simulink library "mympclib"  (R2020a)
settings: Solver=VariableStepAuto  StartTime=0.0  StopTime=10.0  RelTol=1e-3
undefined symbols (not defined in the file): params, sysm, Ts
(part 2 of 2)

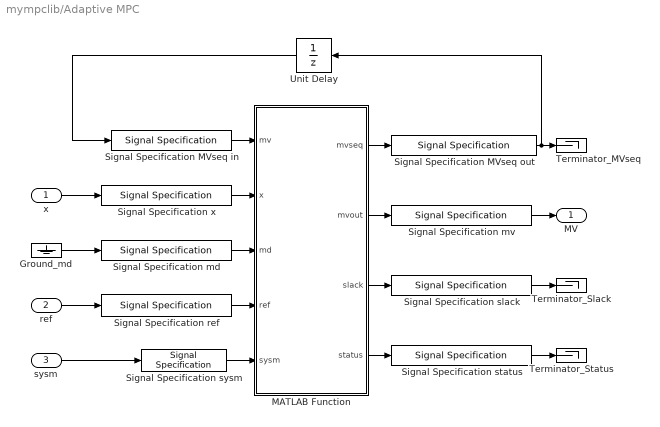
== system mympclib/Adaptive MPC ==
  x : Inport
  ref : Inport  Port=2
  sysm : Inport  Port=3
  Ground_md : Ground
  MATLAB Function : MATLAB Function  TreatAsAtomicUnit=on  SystemSampleTime=Ts
  Signal Specification MVseq in : SignalSpecification  OutDataTypeStr=double  Dimensions=index2  SampleTime=Ts
  Signal Specification MVseq out : SignalSpecification  OutDataTypeStr=double  Dimensions=index2  SampleTime=Ts
  Signal Specification md : SignalSpecification  OutDataTypeStr=double  Dimensions=numDist  SampleTime=Ts
  Signal Specification mv : SignalSpecification  OutDataTypeStr=double  Dimensions=numMV  SampleTime=Ts
  Signal Specification ref : SignalSpecification  OutDataTypeStr=double  Dimensions=numRef  SampleTime=Ts
  Signal Specification slack : SignalSpecification  OutDataTypeStr=double  Dimensions=1  SampleTime=Ts
  Signal Specification status : SignalSpecification  OutDataTypeStr=boolean  Dimensions=1  SampleTime=Ts
  Signal Specification sysm : SignalSpecification  SampleTime=Ts
  Signal Specification x : SignalSpecification  OutDataTypeStr=double  Dimensions=numState  SampleTime=Ts
  Terminator_MVseq : Terminator
  Terminator_Slack : Terminator
  Terminator_Status : Terminator
  Unit Delay : UnitDelay  InitialCondition=kron(ones(params.ControlHorizon,1) , params.initialconditionMV)  SampleTime=-1  HasFrameUpgradeWarning=on
  MV : Outport
  wires:
  MATLAB Function/3(slack) -> Signal Specification slack/1
  MATLAB Function/4(status) -> Signal Specification status/1
  x/1 -> Signal Specification x/1
  ref/1 -> Signal Specification ref/1
  Signal Specification x/1 -> MATLAB Function/2(x)
  Signal Specification md/1 -> MATLAB Function/3(md)
  Signal Specification ref/1 -> MATLAB Function/4(ref)
  sysm/1 -> Signal Specification sysm/1
  MATLAB Function/2(mvout) -> Signal Specification mv/1
  Signal Specification sysm/1 -> MATLAB Function/5(sysm)
  MATLAB Function/1(mvseq) -> Signal Specification MVseq out/1
  Unit Delay/1 -> Signal Specification MVseq in/1
  Signal Specification mv/1 -> MV/1
  Signal Specification MVseq in/1 -> MATLAB Function/1(mv)
  Signal Specification MVseq out/1 -> Unit Delay/1, Terminator_MVseq/1
  Signal Specification slack/1 -> Terminator_Slack/1
  Signal Specification status/1 -> Terminator_Status/1
  Ground_md/1 -> Signal Specification md/1

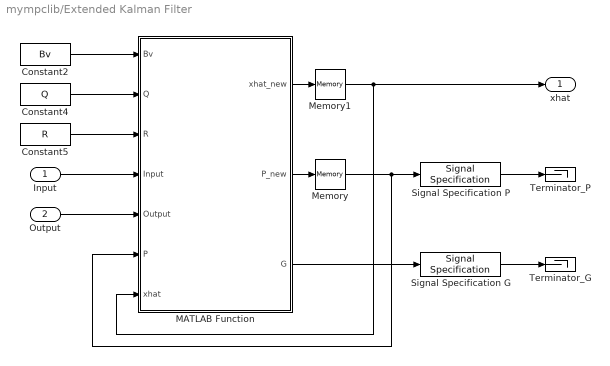
== system mympclib/Extended Kalman Filter ==
  Input : Inport
  Output : Inport  Port=2
  Constant2 : Constant  Value=Bv
  Constant4 : Constant  Value=Q
  Constant5 : Constant  Value=R
  MATLAB Function : MATLAB Function  TreatAsAtomicUnit=on  SystemSampleTime=Ts
  Memory : Memory  InitialCondition=P0  InheritSampleTime=on  LinearizeMemory=on  LinearizeAsDelay=on
  Memory1 : Memory  InitialCondition=xhat0  InheritSampleTime=on  LinearizeMemory=on  LinearizeAsDelay=on
  Signal Specification G : SignalSpecification  SampleTime=Ts
  Signal Specification P : SignalSpecification  SampleTime=Ts
  Terminator_G : Terminator
  Terminator_P : Terminator
  xhat : Outport
  wires:
  Constant2/1 -> MATLAB Function/1(Bv)
  MATLAB Function/3(G) -> Signal Specification G/1
  Constant5/1 -> MATLAB Function/3(R)
  Memory1/1 -> xhat/1, MATLAB Function/7(xhat)
  MATLAB Function/2(P_new) -> Memory/1
  MATLAB Function/1(xhat_new) -> Memory1/1
  Input/1 -> MATLAB Function/4(Input)
  Output/1 -> MATLAB Function/5(Output)
  Constant4/1 -> MATLAB Function/2(Q)
  Memory/1 -> Signal Specification P/1, MATLAB Function/6(P)
  Signal Specification P/1 -> Terminator_P/1
  Signal Specification G/1 -> Terminator_G/1

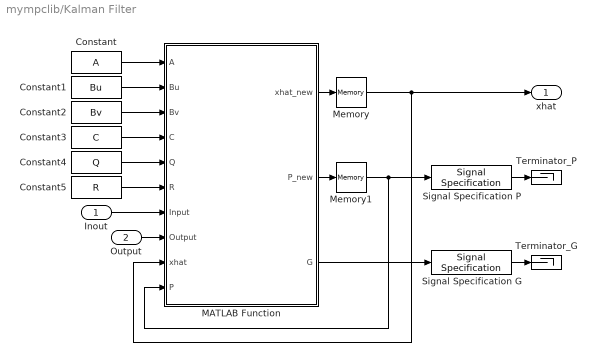
== system mympclib/Kalman Filter ==
  Inout : Inport
  Output : Inport  Port=2
  Constant : Constant  Value=A
  Constant1 : Constant  Value=Bu
  Constant2 : Constant  Value=Bv
  Constant3 : Constant  Value=C
  Constant4 : Constant  Value=Q
  Constant5 : Constant  Value=R
  MATLAB Function : MATLAB Function  TreatAsAtomicUnit=on  SystemSampleTime=Ts
  Memory : Memory  InitialCondition=xhat0  InheritSampleTime=on  LinearizeMemory=on  LinearizeAsDelay=on
  Memory1 : Memory  InitialCondition=P0  InheritSampleTime=on  LinearizeMemory=on  LinearizeAsDelay=on
  Signal Specification G : SignalSpecification  SampleTime=Ts
  Signal Specification P : SignalSpecification  SampleTime=Ts
  Terminator_G : Terminator
  Terminator_P : Terminator
  xhat : Outport
  wires:
  MATLAB Function/3(G) -> Signal Specification G/1
  Constant1/1 -> MATLAB Function/2(Bu)
  MATLAB Function/2(P_new) -> Memory1/1
  MATLAB Function/1(xhat_new) -> Memory/1
  Constant5/1 -> MATLAB Function/6(R)
  Inout/1 -> MATLAB Function/7(Input)
  Constant2/1 -> MATLAB Function/3(Bv)
  Constant3/1 -> MATLAB Function/4(C)
  Constant/1 -> MATLAB Function/1(A)
  Output/1 -> MATLAB Function/8(Output)
  Constant4/1 -> MATLAB Function/5(Q)
  Memory/1 -> MATLAB Function/9(xhat), xhat/1
  Memory1/1 -> MATLAB Function/10(P), Signal Specification P/1
  Signal Specification P/1 -> Terminator_P/1
  Signal Specification G/1 -> Terminator_G/1

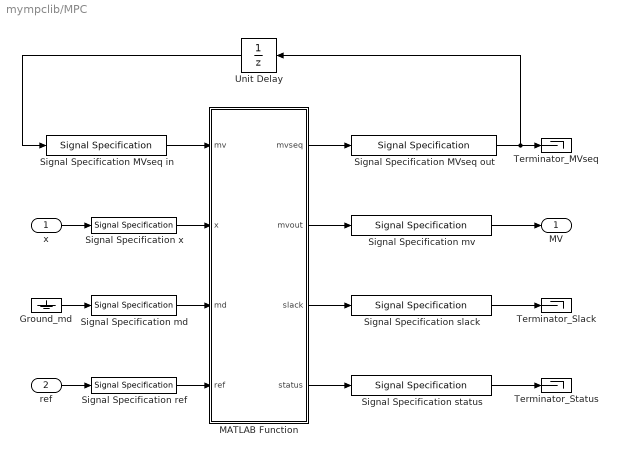
== system mympclib/MPC ==
  x : Inport
  ref : Inport  Port=2
  Ground_md : Ground
  MATLAB Function : MATLAB Function  TreatAsAtomicUnit=on  SystemSampleTime=Ts
  Signal Specification MVseq in : SignalSpecification  OutDataTypeStr=double  Dimensions=index2  SampleTime=Ts
  Signal Specification MVseq out : SignalSpecification  OutDataTypeStr=double  Dimensions=index2  SampleTime=Ts
  Signal Specification md : SignalSpecification  Dimensions=numDist  SampleTime=Ts
  Signal Specification mv : SignalSpecification  OutDataTypeStr=double  Dimensions=numMV  SampleTime=Ts
  Signal Specification ref : SignalSpecification  Dimensions=numRef  SampleTime=Ts
  Signal Specification slack : SignalSpecification  OutDataTypeStr=double  Dimensions=1  SampleTime=Ts
  Signal Specification status : SignalSpecification  OutDataTypeStr=boolean  Dimensions=1  SampleTime=Ts
  Signal Specification x : SignalSpecification  Dimensions=numState  SampleTime=Ts
  Terminator_MVseq : Terminator
  Terminator_Slack : Terminator
  Terminator_Status : Terminator
  Unit Delay : UnitDelay  InitialCondition=kron(ones(params.ControlHorizon,1) , params.initialconditionMV)  SampleTime=-1  HasFrameUpgradeWarning=on
  MV : Outport
  wires:
  Signal Specification ref/1 -> MATLAB Function/4(ref)
  Signal Specification md/1 -> MATLAB Function/3(md)
  Signal Specification x/1 -> MATLAB Function/2(x)
  ref/1 -> Signal Specification ref/1
  x/1 -> Signal Specification x/1
  MATLAB Function/4(status) -> Signal Specification status/1
  MATLAB Function/3(slack) -> Signal Specification slack/1
  MATLAB Function/2(mvout) -> Signal Specification mv/1
  Signal Specification MVseq in/1 -> MATLAB Function/1(mv)
  MATLAB Function/1(mvseq) -> Signal Specification MVseq out/1
  Signal Specification mv/1 -> MV/1
  Signal Specification MVseq out/1 -> Unit Delay/1, Terminator_MVseq/1
  Unit Delay/1 -> Signal Specification MVseq in/1
  Ground_md/1 -> Signal Specification md/1
  Signal Specification slack/1 -> Terminator_Slack/1
  Signal Specification status/1 -> Terminator_Status/1

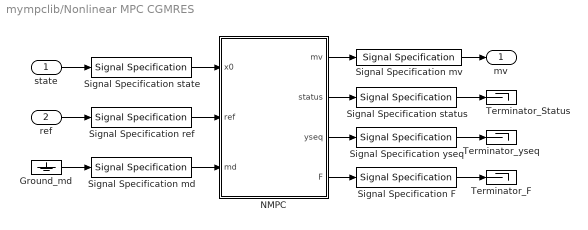
== system mympclib/Nonlinear MPC CGMRES ==
  state : Inport
  ref : Inport  Port=2
  Ground_md : Ground
  NMPC : MATLAB Function  TreatAsAtomicUnit=on  SystemSampleTime=Ts
  Signal Specification F : SignalSpecification  OutDataTypeStr=double  Dimensions=1  SampleTime=Ts
  Signal Specification md : SignalSpecification  OutDataTypeStr=double  Dimensions=nd  SampleTime=Ts
  Signal Specification mv : SignalSpecification  OutDataTypeStr=double  Dimensions=nmv  SampleTime=Ts
  Signal Specification ref : SignalSpecification  OutDataTypeStr=double  Dimensions=nx  SampleTime=Ts
  Signal Specification state : SignalSpecification  OutDataTypeStr=double  Dimensions=nx  SampleTime=Ts
  Signal Specification status : SignalSpecification  OutDataTypeStr=boolean  Dimensions=1  SampleTime=Ts
  Signal Specification yseq : SignalSpecification  OutDataTypeStr=double  Dimensions=nyseq  SampleTime=Ts
  Terminator_F : Terminator
  Terminator_Status : Terminator
  Terminator_yseq : Terminator
  mv : Outport
  wires:
  NMPC/1(mv) -> Signal Specification mv/1
  NMPC/2(status) -> Signal Specification status/1
  state/1 -> Signal Specification state/1
  ref/1 -> Signal Specification ref/1
  Signal Specification state/1 -> NMPC/1(x0)
  Signal Specification ref/1 -> NMPC/2(ref)
  Signal Specification md/1 -> NMPC/3(md)
  Signal Specification mv/1 -> mv/1
  NMPC/3(yseq) -> Signal Specification yseq/1
  NMPC/4(F) -> Signal Specification F/1
  Ground_md/1 -> Signal Specification md/1
  Signal Specification yseq/1 -> Terminator_yseq/1
  Signal Specification status/1 -> Terminator_Status/1
  Signal Specification F/1 -> Terminator_F/1

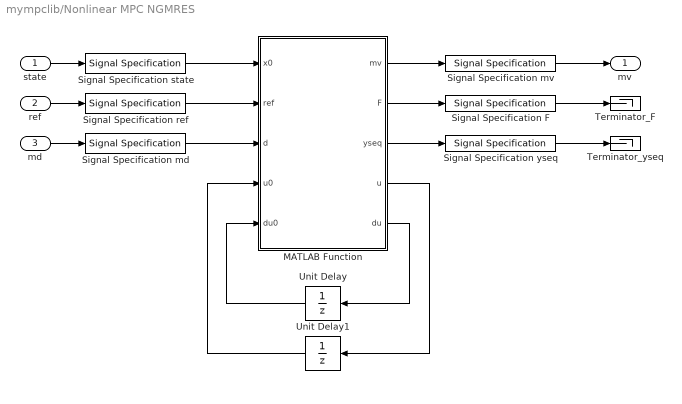
== system mympclib/Nonlinear MPC NGMRES ==
  state : Inport
  ref : Inport  Port=2
  md : Inport  Port=3
  MATLAB Function : MATLAB Function  TreatAsAtomicUnit=on  SystemSampleTime=Ts
  Signal Specification F : SignalSpecification  OutDataTypeStr=double  Dimensions=1  SampleTime=Ts
  Signal Specification md : SignalSpecification  OutDataTypeStr=double  Dimensions=nd  SampleTime=Ts
  Signal Specification mv : SignalSpecification  OutDataTypeStr=double  Dimensions=nmv  SampleTime=Ts
  Signal Specification ref : SignalSpecification  OutDataTypeStr=double  Dimensions=nx  SampleTime=Ts
  Signal Specification state : SignalSpecification  OutDataTypeStr=double  Dimensions=nx  SampleTime=Ts
  Signal Specification yseq : SignalSpecification  OutDataTypeStr=double  Dimensions=nyseq  SampleTime=Ts
  Terminator_F : Terminator
  Terminator_yseq : Terminator
  Unit Delay : UnitDelay  InitialCondition=du0  SampleTime=Ts  HasFrameUpgradeWarning=on
  Unit Delay1 : UnitDelay  InitialCondition=u0  SampleTime=Ts  HasFrameUpgradeWarning=on
  mv : Outport
  wires:
  MATLAB Function/3(yseq) -> Signal Specification yseq/1
  Signal Specification md/1 -> MATLAB Function/3(d)
  Signal Specification ref/1 -> MATLAB Function/2(ref)
  Signal Specification state/1 -> MATLAB Function/1(x0)
  Signal Specification mv/1 -> mv/1
  MATLAB Function/2(F) -> Signal Specification F/1
  Unit Delay/1 -> MATLAB Function/5(du0)
  state/1 -> Signal Specification state/1
  MATLAB Function/4(u) -> Unit Delay1/1
  Unit Delay1/1 -> MATLAB Function/4(u0)
  ref/1 -> Signal Specification ref/1
  MATLAB Function/1(mv) -> Signal Specification mv/1
  MATLAB Function/5(du) -> Unit Delay/1
  md/1 -> Signal Specification md/1
  Signal Specification yseq/1 -> Terminator_yseq/1
  Signal Specification F/1 -> Terminator_F/1

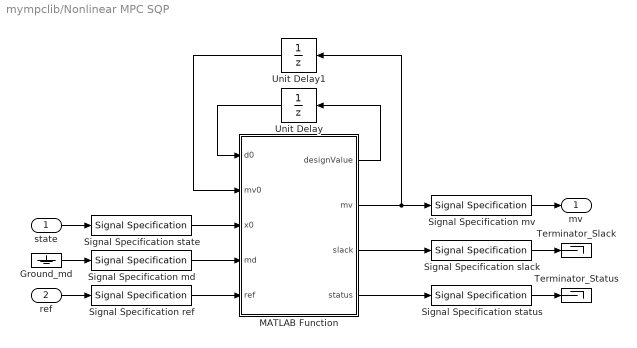
== system mympclib/Nonlinear MPC SQP ==
  state : Inport
  ref : Inport  Port=2
  Ground_md : Ground
  MATLAB Function : MATLAB Function  TreatAsAtomicUnit=on  SystemSampleTime=Ts
  Signal Specification md : SignalSpecification  OutDataTypeStr=double  Dimensions=nd  SampleTime=Ts
  Signal Specification mv : SignalSpecification  OutDataTypeStr=double  Dimensions=nu  SampleTime=Ts
  Signal Specification ref : SignalSpecification  OutDataTypeStr=double  Dimensions=ny  SampleTime=Ts
  Signal Specification slack : SignalSpecification  OutDataTypeStr=double  Dimensions=1  SampleTime=Ts
  Signal Specification state : SignalSpecification  OutDataTypeStr=double  Dimensions=nx  SampleTime=Ts
  Signal Specification status : SignalSpecification  OutDataTypeStr=boolean  Dimensions=1  SampleTime=Ts
  Terminator_Slack : Terminator
  Terminator_Status : Terminator
  Unit Delay : UnitDelay  InitialCondition=d0  SampleTime=Ts  HasFrameUpgradeWarning=on
  Unit Delay1 : UnitDelay  InitialCondition=mv0  SampleTime=Ts  HasFrameUpgradeWarning=on
  mv : Outport
  wires:
  state/1 -> Signal Specification state/1
  MATLAB Function/2(mv) -> Signal Specification mv/1, Unit Delay1/1
  MATLAB Function/1(designValue) -> Unit Delay/1
  Unit Delay/1 -> MATLAB Function/1(d0)
  ref/1 -> Signal Specification ref/1
  MATLAB Function/4(status) -> Signal Specification status/1
  MATLAB Function/3(slack) -> Signal Specification slack/1
  Unit Delay1/1 -> MATLAB Function/2(mv0)
  Signal Specification state/1 -> MATLAB Function/3(x0)
  Signal Specification md/1 -> MATLAB Function/4(md)
  Signal Specification ref/1 -> MATLAB Function/5(ref)
  Signal Specification mv/1 -> mv/1
  Ground_md/1 -> Signal Specification md/1
  Signal Specification slack/1 -> Terminator_Slack/1
  Signal Specification status/1 -> Terminator_Status/1

== matlab function mympclib/Nonlinear MPC SQP/MATLAB Function ==
  data: d0 input; mv0 input; designValue output; x0 input; md input; ref input; mv output; slack output; status output; params parameter; ny parameter; nu parameter; nx parameter
function [designValue,mv,slack,status] = fcn(d0,mv0,x0,md,ref,params,ny,nu,nx)
% Wraper for the nmpcfcn

% Initialization
designValue = zeros(length(d0),1,'like',d0);
mv = zeros(length(mv0),1,'like',mv0);
slack = zeros(1);
status = false;

[designValue,mv,slack,status] = nmpcfcn(d0,x0,mv0,md,ref,params,ny,nu,nx);
end
%EOF

== matlab function mympclib/Nonlinear MPC CGMRES/NMPC ==
  data: x0 input; mv output; ref input; md input; params parameter; status output; nmv parameter; Ts parameter; yseq output; F output
function [mv,status,yseq,F] = CGMRES(x0,ref,md,params,nmv,Ts)
%#codegen
% Wrapper function for cgmresfcn  
% 
% Arguments
% x0:Intial State
% ref:Refernce value of state
% md:Measurement Disturbance
% params:Parameter Structure
% nmv:Number of mv
% 
% Outputs
% mv:Manipulated Variable
% status:Optimization Flag True or False
% yseq:Predictive output sequence 
% F:L2 norm of aglebraic eqn

% Permanent variables
persistent flag;
persistent u;
persistent du;
persistent T;

% Initilization
mv = zeros(nmv,1);
status = false;
yseq = zeros(length(x0),params.divideNumber);
F = Inf;

% Initialization
len_u = length(params.initialConditionInputs);
model = str2func(params.stateFunction);             % Function handle for the state function
dPhidx = str2func(params.jacobianTerminalFunction); % Function handle for the Jacobian of the terminal function phi
dHdx = str2func(params.jacobianHamiltonianState);   % Function handle for the Jacobian of the hamiltonian function H about state
dHdu = str2func(params.jacobianHamiltonianInput);   % Function handle for the Jacobian of the hamiltonian function H about input

if isempty(flag)
    flag = false;
end
if isempty(du)
    du = zeros(len_u*params.divideNumber,1);
end
if isempty(u)
    u = zeros(len_u*params.divideNumber,1);
end
if isempty(T)
    T = 0;
end
if ~flag
    du = repmat(params.initialConditionInputs,params.divideNumber,1);
    u = du;
    flag = true;
end

% Solve optimization problem by CGMRES method
[duopt,status] = cgmresfcn(x0,u,du,md,ref,T,params);
if status
    du = duopt;
    u = u + du*Ts;                          % Integrating mv
end

% Output mv value
mv = u(1:nmv);

% Calc yseq
nx = length(x0);
nu = 1:len_u;
x = x0;
for i = 1:params.divideNumber
     utemp = u(nu);
     x = model(x,utemp(1:nmv),md);
     yseq(1:nx,i) = x;
     nu = nu + len_u;
end

% F L2norm
ts = T/params.divideNumber;
F = norm(calcDiff(x0,u,md,ref,ts,params,model,dPhidx,dHdx,dHdu));

% Increasing predicition time as first order delay
T = params.T_a*T + params.T_b;    
end

== matlab function mympclib/Nonlinear MPC NGMRES/MATLAB Function ==
  data: mv output; F output; yseq output; u output; x0 input; ref input; d input; du output; u0 input; du0 input; params parameter; nmv parameter
function [mv,F,yseq,u,du] = ngmresfcn(x0,ref,d,u0,du0,params,nmv)
%#codegen
% This is the NMPC function by using Newton-GMRES method 
% 
% Arguments
% x0:Intial State [n,1]
% u0:Previous Input [nu*divideTime,1]
% du0:Previous rate of input [nu*divideTime,1]
% d:Disturbance [nd,1]
% ref:Refernce value of state [ny,1]
% T:Prediction time Scalar
% params:Parameter Structure
% nmv:Number of manipulated variable
% 
% Outputs
% du:Rate of input [nu*divideTime,1]
% u:Input [nu*divideTime,1]
% mv:Manipulated variable

persistent T;

if isempty(T)
    T = 0;
end

% Initialization
du = zeros(length(du0),1,'like',du0);
u = zeros(length(u0),1,'like',u0);
len_u = length(params.initialConditionInputs);
mv = zeros(nmv,1);
yseq = zeros(length(x0),params.divideNumber);
max_iter = params.OuterIterationMax;
ts = T/params.divideNumber;                         % Sampling time during current prediction time
model = str2func(params.stateFunction);             % Function handle for the state function
dPhidx = str2func(params.jacobianTerminalFunction); % Function handle for the Jacobian of the terminal function phi
dHdx = str2func(params.jacobianHamiltonianState);   % Function handle for the Jacobian of the hamiltonian function H about state
dHdu = str2func(params.jacobianHamiltonianInput);   % Function handle for the Jacobian of the hamiltonian function H about input

% Newton-GMRES Loop
f0 = calcDiff(x0,u0,d,ref,ts,params,model,dPhidx,dHdx,dHdu);
du = fdgmres(f0,x0,u0,d,ref,du0,ts,params,model,dPhidx,dHdx,dHdu);
u = u0 + du;
for i = 1:max_iter
    f0 = calcDiff(x0,u,d,ref,ts,params,model,dPhidx,dHdx,dHdu);
    du = fdgmres(f0,x0,u,d,ref,du,ts,params,model,dPhidx,dHdx,dHdu);
    u = u + du;
end

% Extract first element from input vector
mv = u(1:nmv);

% Norm of nonlinerar algebraic vector
F = norm(calcDiff(x0,u,d,ref,ts,params,model,dPhidx,dHdx,dHdu));

% Calc yseq
nx = length(x0);
nu = 1:len_u;
x = x0;
for i = 1:params.divideNumber
     utemp = u(nu);
     x = model(x,utemp(1:nmv),d);
     yseq(1:nx,i) = x;
     nu = nu + len_u;
end

% Increasing predictive time
T = params.T_a * T + params.T_b;

end
%EOF

== matlab function mympclib/Kalman Filter/MATLAB Function ==
  data: A input; xhat_new output; Bu input; Bv input; C input; Q input; R input; Input input; Output input; xhat input; P input; P_new output; G output
function [xhat_new,P_new,G] = fcn(A,Bu,Bv,C,Q,R,Input,Output,xhat,P)
%#codegen
% Wrapper function for Kalman filter function kf

% Initialization
n = size(A,1);
l = length(Output);
xhat_new = zeros(n,1);
P_new = zeros(n);
G = zeros(n,l);

% Call kf fucntion
[xhat_new,P_new,G] = kf(A,Bu,Bv,C,Q,R,Input,Output,xhat,P);
end
%EOF

== matlab function mympclib/MPC/MATLAB Function ==
  data: mvseq output; mv input; x input; mvout output; md input; ref input; slack output; status output boolean; params parameter; sysm parameter; index parameter size=1; index2 parameter size=1; index3 parameter size=1; index4 parameter size=1; index5 parameter size=1
function [mvseq,mvout,slack,status] = fcn(mv,x,md,ref,params,sysm,index,index2,index3,index4,index5)
% Wrapper of "mpcfcn"
% x:Output value(OV)
% d:Disturbance
% ref:Reference for OV
% sysm:Construnstion of system(A,B,C,D)
% params:MPC parameter constructs
% Dimenstions of each matrix:
% index = n*Hp
% index2 = m*Hc
% index3 = l*Hp
% index4 = (m*Hc)+1
% index5 = (4*index2)+(2*index3)+1
% Initlialization of outputs

% coder.extrinsic('mpcfcn');

% Initlialization of outputs
m = size(sysm.B,2);
slack = zeros(1);
status = false;
mvseq = zeros(index2,1);
mvout = zeros(m,1);

% Call mpcfcn
[mvopt,slack,status] = mpcfcn(x,mv,md,ref,sysm,params,index,index2,index3,index4,index5);
mvout = mvopt(1:m,1);
mvseq = mvopt;
%EOF

== matlab function mympclib/Adaptive MPC/MATLAB Function ==
  data: mvseq output; mv input; x input; mvout output; md input; ref input; slack output; status output boolean; params parameter; sysm input; index parameter size=1; index2 parameter size=1; index3 parameter size=1; index4 parameter size=1; index5 parameter size=1
function [mvseq,mvout,slack,status] = fcn(mv,x,md,ref,params,sysm,index,index2,index3,index4,index5)
% Wrapper of "mpcfcn"
% x:Output value(OV)
% d:Disturbance
% ref:Reference for OV
% sysm:Construnstion of system(A,B,C,D)
% params:MPC parameter constructs
% Dimenstions of each matrix:
% index = n*Hp
% index2 = m*Hc
% index3 = l*Hp
% index4 = (m*Hc)+1
% index5 = (4*index2)+(2*index3)+1

% Initlialization of outputs
m = size(sysm.B,2);
slack = zeros(1);
status = false;
mvseq = zeros(index2,1);
mvout = zeros(m,1);

% Call mpcfcn
[mvopt,slack,status] = mpcfcn(x,mv,md,ref,sysm,params,index,index2,index3,index4,index5);
mvout = mvopt(1:m,1);
mvseq = mvopt;
%EOF

== matlab function mympclib/Extended Kalman Filter/MATLAB Function ==
  data: xhat_new output; Bv input; Q input; R input; Input input; Output input; P input; xhat input; P_new output; G output; numState parameter; numOutput parameter; Ts parameter; p parameter
function [xhat_new,P_new,G] = fcn(Bv,Q,R,Input,Output,P,xhat,numState,numOutput,Ts,p)
%#codegen
% Wrapper function for Extended Kalman filter function ekf

% Initialization
n = numState;
l = numOutput;
xhat_new = zeros(n,1);
P_new = zeros(n);
G = zeros(n,l);

% Function handle
f = str2func(p.stateFunction);
h = str2func(p.measurementFunction);
A = str2func(p.jacobianStateFunction);
C = str2func(p.jacobianOfMeasurementFunction);

% Call kf fucntion
[xhat_new,P_new,G] = ekf(f,h,A,C,Bv,Q,R,Input,Output,xhat,P,Ts);
end
%EOF
